simulink model "Sim"  (R2020b)
settings: Solver=VariableStepAuto  StartTime=0.0  StopTime=200.0  MaxStep=0.001  RelTol=1e-10
values from neighbouring files (symbols this model uses):
  Ap = 3.14*Rp*Rp    (= 0.005024)    [Projekt_1.m]
  Az = 3.14*Rz*Rz    (= 3.14)    [Projekt_1.m]
  f = 0.1    [Projekt_1.m]
  g = 9.81    [Projekt_1.m]
  h0 = 0.2    [Projekt_1.m]
  kf = 0.5    [Projekt_1.m]
  L = 1    [Projekt_1.m]
  Qwe = 0.1    [Projekt_1.m]
  ro = 1000    [Projekt_1.m]
  typ_wymuszenia = 2    [Projekt_1.m]
settings Model: Creator=Bartek  LastModifiedBy=Bartek
settings SolverCC: AlgebraicLoopSolver=LineSearch

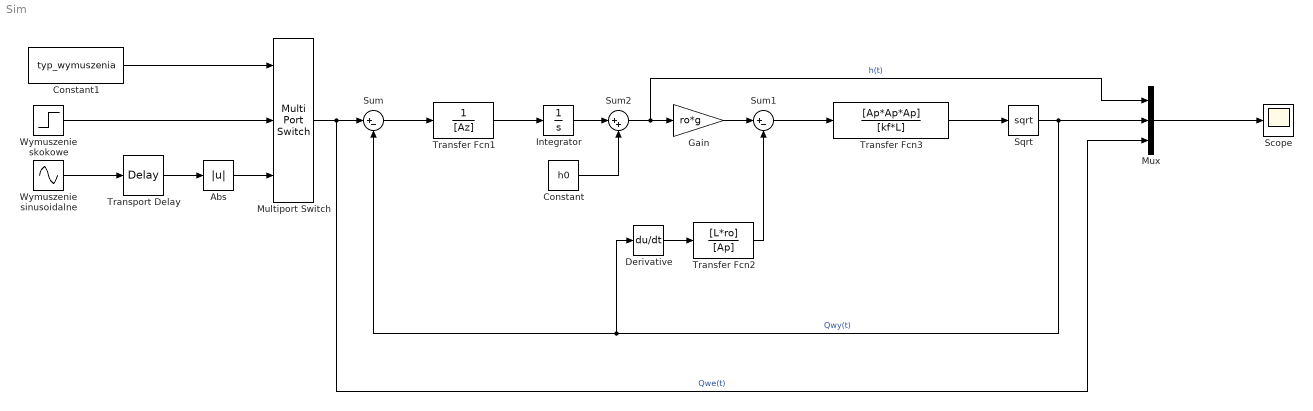
== system Sim ==
  Abs : Abs
  Constant : Constant  Value=h0
  Constant1 : Constant  Value=typ_wymuszenia
  Derivative : Derivative
  Gain : Gain  Gain=ro*g
  Integrator : Integrator
  Multiport Switch : MultiPortSwitch  Inputs=2
  Mux : Mux  Inputs=3
  Scope : Scope
  Sqrt : Sqrt  SaturateOnIntegerOverflow=on
  Sum : Sum  Inputs=|+-
  Sum1 : Sum  Inputs=|+-
  Sum2 : Sum  Inputs=|++
  Transfer Fcn1 : TransferFcn  Denominator=[Az]
  Transfer Fcn2 : TransferFcn  Numerator=[L*ro]  Denominator=[Ap]
  Transfer Fcn3 : TransferFcn  Numerator=[Ap*Ap*Ap]  Denominator=[kf*L]
  Transport Delay : TransportDelay  DelayTime=5
  Wymuszenie sinusoidalne : Sin  Amplitude=Qwe  Frequency=f  SampleTime=0
  Wymuszenie skokowe : Step  Time=5  After=Qwe  SampleTime=0
  wires:
  Sum/1 -> Transfer Fcn1/1
  Integrator/1 -> Sum2/1
  Constant/1 -> Sum2/2
  Sum2/1 -> Gain/1, Mux/1  "h(t)"
  Sum1/1 -> Transfer Fcn3/1
  Sqrt/1 -> Mux/2, Derivative/1, Sum/2  "Qwy(t)"
  Transfer Fcn1/1 -> Integrator/1
  Gain/1 -> Sum1/1
  Wymuszenie skokowe/1 -> Multiport Switch/2
  Constant1/1 -> Multiport Switch/1
  Mux/1 -> Scope/1
  Multiport Switch/1 -> Mux/3, Sum/1  "Qwe(t)"
  Wymuszenie sinusoidalne/1 -> Transport Delay/1
  Transport Delay/1 -> Abs/1
  Abs/1 -> Multiport Switch/3
  Derivative/1 -> Transfer Fcn2/1
  Transfer Fcn3/1 -> Sqrt/1
  Transfer Fcn2/1 -> Sum1/2
